simulink model "p3Sim"  (R2019a)
settings: Solver=ode4  StartTime=0.0  StopTime=s.TFinal  FixedStep=s.Tstep  RelTol=1e-3
undefined symbols (not defined in the file): a, b, D1, D2, D3, g1, kc, tdrb, tdu
libraries: simulink x1
settings Model: Creator=vtaware  LastModifiedBy=vtaware

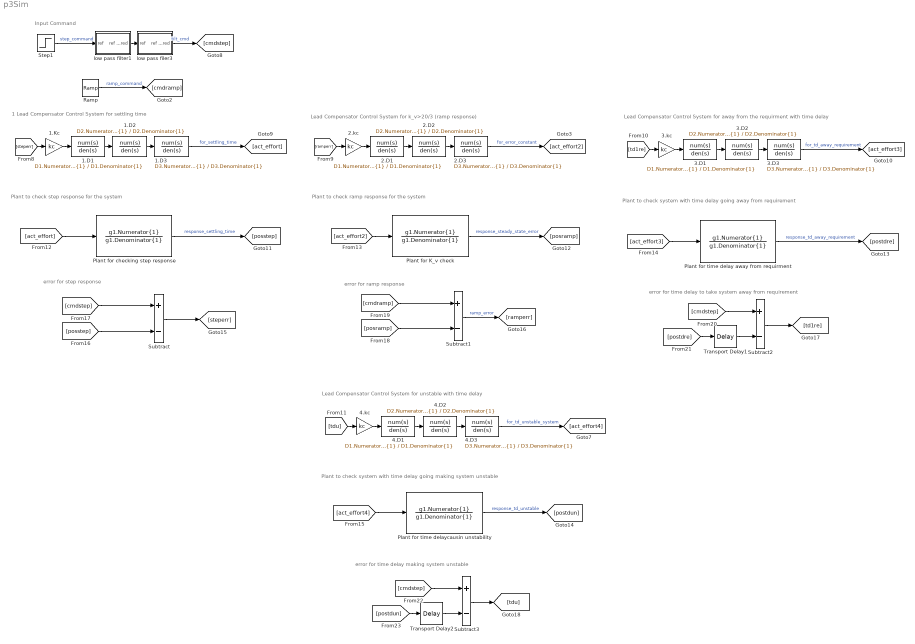
== system p3Sim ==
  note: error for time delay making system unstable
  note: error for time delay to take system away from requirement
  note: error for ramp response
  note: error for step response
  note: Plant to check system with time delay going making system unstable
  note: Plant to check system with time delay going away from requirement
  note: Plant to check ramp response for the system
  note: Plant to check step response for the system
  note: 1 Lead Compensator Control System for settling time
  note: Input Command
  note: Lead Compensator Control System for k_v>20/3 (ramp response)
  note: Lead Compensator Control System for away from the requirment
      | with time delay
  note: Lead Compensator Control System for unstable with time delay
  1.D1 : TransferFcn  Numerator=D1.Numerator{1}  Denominator=D1.Denominator{1}
  1.D2 : TransferFcn  Numerator=D2.Numerator{1}  Denominator=D2.Denominator{1}
  1.D3 : TransferFcn  Numerator=D3.Numerator{1}  Denominator=D3.Denominator{1}
  1.Kc : Gain  Gain=kc
  2.D1 : TransferFcn  Numerator=D1.Numerator{1}  Denominator=D1.Denominator{1}
  2.D2 : TransferFcn  Numerator=D2.Numerator{1}  Denominator=D2.Denominator{1}
  2.D3 : TransferFcn  Numerator=D3.Numerator{1}  Denominator=D3.Denominator{1}
  2.kc : Gain  Gain=kc
  3.D1 : TransferFcn  Numerator=D1.Numerator{1}  Denominator=D1.Denominator{1}
  3.D2 : TransferFcn  Numerator=D2.Numerator{1}  Denominator=D2.Denominator{1}
  3.D3 : TransferFcn  Numerator=D3.Numerator{1}  Denominator=D3.Denominator{1}
  3.kc : Gain  Gain=kc
  4.D1 : TransferFcn  Numerator=D1.Numerator{1}  Denominator=D1.Denominator{1}
  4.D2 : TransferFcn  Numerator=D2.Numerator{1}  Denominator=D2.Denominator{1}
  4.D3 : TransferFcn  Numerator=D3.Numerator{1}  Denominator=D3.Denominator{1}
  4.kc : Gain  Gain=kc
  Plant for K_v check : TransferFcn  Numerator=g1.Numerator{1}  Denominator=g1.Denominator{1}
  Plant for checking step response : TransferFcn  Numerator=g1.Numerator{1}  Denominator=g1.Denominator{1}
  Plant for time delay away from requirment : TransferFcn  Numerator=g1.Numerator{1}  Denominator=g1.Denominator{1}
  Plant for time delaycausin unstability : TransferFcn  Numerator=g1.Numerator{1}  Denominator=g1.Denominator{1}
  Ramp : simulink/Sources/Ramp  slope=b.A  start=b.T0  InitialOutput=0
  Step1 : Step  Time=a.T0  After=a.A  SampleTime=0
  Subtract{,1..3} (4 alike) : Sum  Inputs=+-
  Transport Delay1 : TransportDelay  DelayTime=tdrb
  Transport Delay2 : TransportDelay  DelayTime=tdu
  low pass filer3 : Subsystem  mask{tau=0.15}
  low pass filter1 : Subsystem  mask{tau=0.15}
  wires:
  Step1/1 -> low pass filter1/1(ref)  "step_command"
  low pass filter1/1(ref filtered) -> low pass filer3/1(ref)
  low pass filer3/1(ref filtered) -> [cmdstep]  "filt_cmd"
  Ramp/1 -> [cmdramp]  "ramp_command"
  1.D1/1 -> 1.D2/1
  1.Kc/1 -> 1.D1/1
  [steperr] -> 1.Kc/1
  [ramperr] -> 2.kc/1
  2.kc/1 -> 2.D1/1
  2.D2/1 -> 2.D3/1
  2.D1/1 -> 2.D2/1
  3.D1/1 -> 3.D2/1
  3.kc/1 -> 3.D1/1
  [td1re] -> 3.kc/1
  [tdu] -> 4.kc/1
  4.kc/1 -> 4.D1/1
  4.D1/1 -> 4.D2/1
  [act_effort] -> Plant for checking step response/1
  [act_effort2] -> Plant for K_v check/1
  [act_effort3] -> Plant for time delay away from requirment/1
  [act_effort4] -> Plant for time delaycausin unstability/1
  Plant for checking step response/1 -> [posstep]  "response_settling_time"
  Plant for K_v check/1 -> [posramp]  "response_steady_state_error"
  Plant for time delay away from requirment/1 -> [postdre]  "response_td_away_requirement"
  Plant for time delaycausin unstability/1 -> [postdun]  "response_td_unstable"
  Subtract/1 -> [steperr]
  [posstep] -> Subtract/2
  [cmdstep] -> Subtract/1
  [cmdramp] -> Subtract1/1
  [posramp] -> Subtract1/2
  Subtract1/1 -> [ramperr]  "ramp_error"
  Subtract2/1 -> [td1re]
  [cmdstep] -> Subtract2/1
  Transport Delay1/1 -> Subtract2/2
  [postdre] -> Transport Delay1/1
  [postdun] -> Transport Delay2/1
  Transport Delay2/1 -> Subtract3/2
  [cmdstep] -> Subtract3/1
  Subtract3/1 -> [tdu]
  1.D2/1 -> 1.D3/1
  1.D3/1 -> [act_effort]  "for_settling_time"
  2.D3/1 -> [act_effort2]  "for_error_constant"
  3.D3/1 -> [act_effort3]  "for_td_away_requirement"
  3.D2/1 -> 3.D3/1
  4.D3/1 -> [act_effort4]  "for_td_unstable_system"
  4.D2/1 -> 4.D3/1

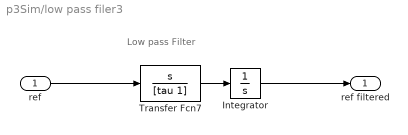
== system p3Sim/low pass filer3 ==
  note: Low pass Filter
  ref : Inport
  Integrator : Integrator
  Transfer Fcn7 : TransferFcn  Numerator=[1 0]  Denominator=[tau 1]
  ref filtered : Outport
  wires:
  Transfer Fcn7/1 -> Integrator/1
  ref/1 -> Transfer Fcn7/1
  Integrator/1 -> ref filtered/1

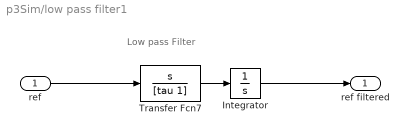
== system p3Sim/low pass filter1 ==
  note: Low pass Filter
  ref : Inport
  Integrator : Integrator
  Transfer Fcn7 : TransferFcn  Numerator=[1 0]  Denominator=[tau 1]
  ref filtered : Outport
  wires:
  Integrator/1 -> ref filtered/1
  ref/1 -> Transfer Fcn7/1
  Transfer Fcn7/1 -> Integrator/1
